simulink library "RF"  (Simulink 4.00)
values from neighbouring files (symbols this model uses):
  A = rms(interp1(f,MX,fb))    [fftbandamp.m]    (also in logfft.m = fftamp(samples, fs, f, varargin{:})/vpp; plotfft.m = fftamp(samples, fs, f, varargin{:})*2/vpp)
  P = sinc((1575.42 - f)/10.23).^2./10.23    [L1PSD.m]    (also in fftphase.m = interp1(f,PX,f0))
undefined symbols (not defined in the file or in its folder): adb, B, CA_ID, fs, j, m, N, p, Phi, Range, Rice_K, Rice_Seed, Rice_Sigma, tau_delay, z
libraries: RF x133, dspcmplx x47, com_sour x8, dspelmat x8, com_chan x4, dspbdsp x3, dspswit x3, simulink_extras x2, com_filt x2
(part 5 of 5)

== system RF/GPS Blocks/C/A Code, 1.023MHz/PN1/1-step delay9 ==
  in_1 : Inport  Port=1
  Constant : Constant  Value=ini
  Constant1 : Constant  Value=n*ts(1)+ts(2)
  Digital Clock : DigitalClock  SampleTime=ts
  K-step delay : DiscreteFilter  Numerator=[zeros(1,n), 1]  Denominator=1  SampleTime=ts  Realization=auto
  Relational Operator : RelationalOperator  Operator=>=
  Switch : Switch  Threshold=.1
  out_1 : Outport  Port=1  InitialOutput=0
  wires:
  Relational Operator/1 -> Switch/2
  Constant1/1 -> Relational Operator/2
  Digital Clock/1 -> Relational Operator/1
  Constant/1 -> Switch/3
  K-step delay/1 -> Switch/1
  in_1/1 -> K-step delay/1
  Switch/1 -> out_1/1

== system RF/GPS Blocks/C/A Code, 1.023MHz/PN2/1-step delay1 ==
  in_1 : Inport  Port=1
  Constant : Constant  Value=ini
  Constant1 : Constant  Value=n*ts(1)+ts(2)
  Digital Clock : DigitalClock  SampleTime=ts
  K-step delay : DiscreteFilter  Numerator=[zeros(1,n), 1]  Denominator=1  SampleTime=ts  Realization=auto
  Relational Operator : RelationalOperator  Operator=>=
  Switch : Switch  Threshold=.1
  out_1 : Outport  Port=1  InitialOutput=0
  wires:
  Relational Operator/1 -> Switch/2
  Constant1/1 -> Relational Operator/2
  Digital Clock/1 -> Relational Operator/1
  Constant/1 -> Switch/3
  K-step delay/1 -> Switch/1
  in_1/1 -> K-step delay/1
  Switch/1 -> out_1/1

== system RF/GPS Blocks/C/A Code, 1.023MHz/PN2/1-step delay10 ==
  in_1 : Inport  Port=1
  Constant : Constant  Value=ini
  Constant1 : Constant  Value=n*ts(1)+ts(2)
  Digital Clock : DigitalClock  SampleTime=ts
  K-step delay : DiscreteFilter  Numerator=[zeros(1,n), 1]  Denominator=1  SampleTime=ts  Realization=auto
  Relational Operator : RelationalOperator  Operator=>=
  Switch : Switch  Threshold=.1
  out_1 : Outport  Port=1  InitialOutput=0
  wires:
  Relational Operator/1 -> Switch/2
  Constant1/1 -> Relational Operator/2
  Digital Clock/1 -> Relational Operator/1
  Constant/1 -> Switch/3
  K-step delay/1 -> Switch/1
  in_1/1 -> K-step delay/1
  Switch/1 -> out_1/1

== system RF/GPS Blocks/C/A Code, 1.023MHz/PN2/1-step delay2 ==
  in_1 : Inport  Port=1
  Constant : Constant  Value=ini
  Constant1 : Constant  Value=n*ts(1)+ts(2)
  Digital Clock : DigitalClock  SampleTime=ts
  K-step delay : DiscreteFilter  Numerator=[zeros(1,n), 1]  Denominator=1  SampleTime=ts  Realization=auto
  Relational Operator : RelationalOperator  Operator=>=
  Switch : Switch  Threshold=.1
  out_1 : Outport  Port=1  InitialOutput=0
  wires:
  Relational Operator/1 -> Switch/2
  Constant1/1 -> Relational Operator/2
  Digital Clock/1 -> Relational Operator/1
  Constant/1 -> Switch/3
  K-step delay/1 -> Switch/1
  in_1/1 -> K-step delay/1
  Switch/1 -> out_1/1

== system RF/GPS Blocks/C/A Code, 1.023MHz/PN2/1-step delay3 ==
  in_1 : Inport  Port=1
  Constant : Constant  Value=ini
  Constant1 : Constant  Value=n*ts(1)+ts(2)
  Digital Clock : DigitalClock  SampleTime=ts
  K-step delay : DiscreteFilter  Numerator=[zeros(1,n), 1]  Denominator=1  SampleTime=ts  Realization=auto
  Relational Operator : RelationalOperator  Operator=>=
  Switch : Switch  Threshold=.1
  out_1 : Outport  Port=1  InitialOutput=0
  wires:
  Relational Operator/1 -> Switch/2
  Constant1/1 -> Relational Operator/2
  Digital Clock/1 -> Relational Operator/1
  Constant/1 -> Switch/3
  K-step delay/1 -> Switch/1
  in_1/1 -> K-step delay/1
  Switch/1 -> out_1/1

== system RF/GPS Blocks/C/A Code, 1.023MHz/PN2/1-step delay4 ==
  in_1 : Inport  Port=1
  Constant : Constant  Value=ini
  Constant1 : Constant  Value=n*ts(1)+ts(2)
  Digital Clock : DigitalClock  SampleTime=ts
  K-step delay : DiscreteFilter  Numerator=[zeros(1,n), 1]  Denominator=1  SampleTime=ts  Realization=auto
  Relational Operator : RelationalOperator  Operator=>=
  Switch : Switch  Threshold=.1
  out_1 : Outport  Port=1  InitialOutput=0
  wires:
  Relational Operator/1 -> Switch/2
  Constant1/1 -> Relational Operator/2
  Digital Clock/1 -> Relational Operator/1
  Constant/1 -> Switch/3
  K-step delay/1 -> Switch/1
  in_1/1 -> K-step delay/1
  Switch/1 -> out_1/1

== system RF/GPS Blocks/C/A Code, 1.023MHz/PN2/1-step delay5 ==
  in_1 : Inport  Port=1
  Constant : Constant  Value=ini
  Constant1 : Constant  Value=n*ts(1)+ts(2)
  Digital Clock : DigitalClock  SampleTime=ts
  K-step delay : DiscreteFilter  Numerator=[zeros(1,n), 1]  Denominator=1  SampleTime=ts  Realization=auto
  Relational Operator : RelationalOperator  Operator=>=
  Switch : Switch  Threshold=.1
  out_1 : Outport  Port=1  InitialOutput=0
  wires:
  Relational Operator/1 -> Switch/2
  Constant1/1 -> Relational Operator/2
  Digital Clock/1 -> Relational Operator/1
  Constant/1 -> Switch/3
  K-step delay/1 -> Switch/1
  in_1/1 -> K-step delay/1
  Switch/1 -> out_1/1

== system RF/GPS Blocks/C/A Code, 1.023MHz/PN2/1-step delay6 ==
  in_1 : Inport  Port=1
  Constant : Constant  Value=ini
  Constant1 : Constant  Value=n*ts(1)+ts(2)
  Digital Clock : DigitalClock  SampleTime=ts
  K-step delay : DiscreteFilter  Numerator=[zeros(1,n), 1]  Denominator=1  SampleTime=ts  Realization=auto
  Relational Operator : RelationalOperator  Operator=>=
  Switch : Switch  Threshold=.1
  out_1 : Outport  Port=1  InitialOutput=0
  wires:
  Relational Operator/1 -> Switch/2
  Constant1/1 -> Relational Operator/2
  Digital Clock/1 -> Relational Operator/1
  Constant/1 -> Switch/3
  K-step delay/1 -> Switch/1
  in_1/1 -> K-step delay/1
  Switch/1 -> out_1/1

== system RF/GPS Blocks/C/A Code, 1.023MHz/PN2/1-step delay7 ==
  in_1 : Inport  Port=1
  Constant : Constant  Value=ini
  Constant1 : Constant  Value=n*ts(1)+ts(2)
  Digital Clock : DigitalClock  SampleTime=ts
  K-step delay : DiscreteFilter  Numerator=[zeros(1,n), 1]  Denominator=1  SampleTime=ts  Realization=auto
  Relational Operator : RelationalOperator  Operator=>=
  Switch : Switch  Threshold=.1
  out_1 : Outport  Port=1  InitialOutput=0
  wires:
  Relational Operator/1 -> Switch/2
  Constant1/1 -> Relational Operator/2
  Digital Clock/1 -> Relational Operator/1
  Constant/1 -> Switch/3
  K-step delay/1 -> Switch/1
  in_1/1 -> K-step delay/1
  Switch/1 -> out_1/1

== system RF/GPS Blocks/C/A Code, 1.023MHz/PN2/1-step delay8 ==
  in_1 : Inport  Port=1
  Constant : Constant  Value=ini
  Constant1 : Constant  Value=n*ts(1)+ts(2)
  Digital Clock : DigitalClock  SampleTime=ts
  K-step delay : DiscreteFilter  Numerator=[zeros(1,n), 1]  Denominator=1  SampleTime=ts  Realization=auto
  Relational Operator : RelationalOperator  Operator=>=
  Switch : Switch  Threshold=.1
  out_1 : Outport  Port=1  InitialOutput=0
  wires:
  Relational Operator/1 -> Switch/2
  Constant1/1 -> Relational Operator/2
  Digital Clock/1 -> Relational Operator/1
  Constant/1 -> Switch/3
  K-step delay/1 -> Switch/1
  in_1/1 -> K-step delay/1
  Switch/1 -> out_1/1

== system RF/GPS Blocks/C/A Code, 1.023MHz/PN2/1-step delay9 ==
  in_1 : Inport  Port=1
  Constant : Constant  Value=ini
  Constant1 : Constant  Value=n*ts(1)+ts(2)
  Digital Clock : DigitalClock  SampleTime=ts
  K-step delay : DiscreteFilter  Numerator=[zeros(1,n), 1]  Denominator=1  SampleTime=ts  Realization=auto
  Relational Operator : RelationalOperator  Operator=>=
  Switch : Switch  Threshold=.1
  out_1 : Outport  Port=1  InitialOutput=0
  wires:
  Relational Operator/1 -> Switch/2
  Constant1/1 -> Relational Operator/2
  Digital Clock/1 -> Relational Operator/1
  Constant/1 -> Switch/3
  K-step delay/1 -> Switch/1
  in_1/1 -> K-step delay/1
  Switch/1 -> out_1/1

== system RF/GPS Blocks/GPS Channel/AWGN channel/Gaussian noise generator1 ==
  Constant : Constant  Value=m
  Matrix Gain : StateSpace  A=[]  B=[]  C=[]  D=K  X0=0  Realization=auto  AbsoluteTolerance=auto  mask(Matrix Gain){@1=d}
      mask prompts: @1 "Gain matrix:"
      mask help: Matrix Gain.
      mask init:
      | K = @1;
      mask Help: Multiplies input vector by entered matrix to produce output vector (y=Au).
      mask Display: disp('K')
  Random Number : RandomNumber  Mean=0  Variance=1  Seed=s  SampleTime=-1
  Sum : Sum  Inputs=++  SaturateOnIntegerOverflow=on
  out_1 : Outport  Port=1  InitialOutput=0
  wires:
  Constant/1 -> Sum/1
  Random Number/1 -> Matrix Gain/1
  Matrix Gain/1 -> Sum/2
  Sum/1 -> out_1/1

== system RF/GPS Blocks/GPS Transmitter/BPSK mod, 1575MHz1/MPSK map ==
  in_1 : Inport  Port=1
  Multiple factor : Constant  Value=Sft
  Product : Product  Inputs=2  Multiplication=Element-wise(.*)  SaturateOnIntegerOverflow=on
  Zero-Order Hold1 : ZeroOrderHold  SampleTime=td
  out_1 : Outport  Port=1  InitialOutput=0
  wires:
  Zero-Order Hold1/1 -> Product/1
  in_1/1 -> Zero-Order Hold1/1
  Product/1 -> out_1/1
  Multiple factor/1 -> Product/2

== system RF/GPS Blocks/GPS Transmitter/BPSK mod, 1575MHz1/PM passband ==
  in_1 : Inport  Port=1  SampleTime=ts
  Clock : Clock
      settings: DisplayTime=off  Decimation=10
  Fcn : Fcn  Expr=cos(u[1])
  Gain : Gain  Gain=Fc  Multiplication=Element-wise(K.*u)  SaturateOnIntegerOverflow=on
  Initial value : Constant  Value=Ph
  Sum1 : Sum  Inputs=+++  SaturateOnIntegerOverflow=on
  Sum2 : Sum  Inputs=+-  SaturateOnIntegerOverflow=on
  Zero-Order Hold : ZeroOrderHold  SampleTime=td
  out_1 : Outport  Port=1  InitialOutput=0
  wires:
  Fcn/1 -> out_1/1
  Initial value/1 -> Sum1/3
  Sum1/1 -> Fcn/1
  in_1/1 -> Sum1/1
  Clock/1 -> Gain/1
  Sum2/1 -> Sum1/2
  Zero-Order Hold/1 -> Sum2/2
  Gain/1 -> Sum2/1, Zero-Order Hold/1

== system RF/GPS Blocks/GPS Transmitter/BPSK mod, 1575MHz2/MPSK map ==
  in_1 : Inport  Port=1
  Multiple factor : Constant  Value=Sft
  Product : Product  Inputs=2  Multiplication=Element-wise(.*)  SaturateOnIntegerOverflow=on
  Zero-Order Hold1 : ZeroOrderHold  SampleTime=td
  out_1 : Outport  Port=1  InitialOutput=0
  wires:
  Zero-Order Hold1/1 -> Product/1
  in_1/1 -> Zero-Order Hold1/1
  Product/1 -> out_1/1
  Multiple factor/1 -> Product/2

== system RF/GPS Blocks/GPS Transmitter/BPSK mod, 1575MHz2/PM passband ==
  in_1 : Inport  Port=1  SampleTime=ts
  Clock : Clock
      settings: DisplayTime=off  Decimation=10
  Fcn : Fcn  Expr=cos(u[1])
  Gain : Gain  Gain=Fc  Multiplication=Element-wise(K.*u)  SaturateOnIntegerOverflow=on
  Initial value : Constant  Value=Ph
  Sum1 : Sum  Inputs=+++  SaturateOnIntegerOverflow=on
  Sum2 : Sum  Inputs=+-  SaturateOnIntegerOverflow=on
  Zero-Order Hold : ZeroOrderHold  SampleTime=td
  out_1 : Outport  Port=1  InitialOutput=0
  wires:
  Fcn/1 -> out_1/1
  Initial value/1 -> Sum1/3
  Sum1/1 -> Fcn/1
  in_1/1 -> Sum1/1
  Clock/1 -> Gain/1
  Sum2/1 -> Sum1/2
  Zero-Order Hold/1 -> Sum2/2
  Gain/1 -> Sum2/1, Zero-Order Hold/1

== system RF/GPS Blocks/GPS Transmitter/P Code, 10.23MHz/P Code, 10.23MHz ==
  Uniform number : S-Function  FunctionName=srandint  Parameters=seed,mul  PortCounts=[]  SFunctionModules=''
  out_1 : Outport  Port=1  InitialOutput=0
  wires:
  Uniform number/1 -> out_1/1

== system RF/Transmission  Channel Blocks/Doppler Fading Envelope/FFT Filter4/Buffer ==
  in_1 : Inport  Port=1
  Buffer : S-Function  FunctionName=sbufferc  Parameters=N,V,Ts,ic  PortCounts=[]  SFunctionModules=''
  ZOH : S-Function  FunctionName=szoh  Parameters=Ts*(N-V)  PortCounts=[]  SFunctionModules=''
  Zero-Order Hold : ZeroOrderHold  SampleTime=Ts
  Outport : Outport  Port=1  InitialOutput=0
  wires:
  Zero-Order Hold/1 -> Buffer/1
  in_1/1 -> Zero-Order Hold/1
  ZOH/1 -> Outport/1
  Buffer/1 -> ZOH/1

== system RF/Transmission  Channel Blocks/Doppler Fading Envelope/FFT Filter4/Complex Multiply1 ==
  note: R = Real
      | I = Imaginary
  Complex input 1 : Inport  Port=1
  Complex input 2 : Inport  Port=2
  Join : dspcmplx/Join
  Product{,1..3} (4 alike) : Product  Inputs=2  Multiplication=Element-wise(.*)  SaturateOnIntegerOverflow=on
  Split : dspcmplx/Split
  Split1 : dspcmplx/Split
  Sum : Sum  Inputs=+-  SaturateOnIntegerOverflow=on
  Sum1 : Sum  Inputs=++  SaturateOnIntegerOverflow=on
  Complex Multiply Result : Outport  Port=1  InitialOutput=0
  wires:
  Product2/1 -> Sum1/2
  Product3/1 -> Sum1/1
  Split/2 -> Product1/1, Product2/2  "I1"
  Split1/2 -> Product1/2, Product3/2  "I2"
  Split1/1 -> Product/2, Product2/1  "R2"
  Split/1 -> Product/1, Product3/1  "R1"
  Product1/1 -> Sum/2
  Product/1 -> Sum/1
  Complex input 2/1 -> Split1/1
  Complex input 1/1 -> Split/1
  Sum/1 -> Join/1  "Rout"
  Sum1/1 -> Join/2  "Iout"
  Join/1 -> Complex Multiply Result/1

== system RF/Transmission  Channel Blocks/Doppler Fading Envelope/FFT Filter4/Filter Response ==
  Complex Constant : Constant  Value=C
  Out1 : Outport  Port=1  InitialOutput=0
  wires:
  Complex Constant/1 -> Out1/1

== system RF/Transmission  Channel Blocks/Doppler Fading Envelope/FFT Filter4/Partial Unbuffer ==
  in_1 : Inport  Port=1
  Complete Unbuffer : S-Function  FunctionName=sunbuffc  Parameters=num_chans,Ts  PortCounts=[]  SFunctionModules=''
  Selector : Selector  InputType=Vector  ElementSrc=Internal  Elements=elements  RowSrc=Internal  Rows=1  ColumnSrc=Internal  Columns=1  InputPortWidth=N*num_chans
  ZOH : S-Function  FunctionName=szoh  Parameters=Ts  PortCounts=[]  SFunctionModules=''
  out_1 : Outport  Port=1  InitialOutput=0
  wires:
  in_1/1 -> Selector/1
  Selector/1 -> ZOH/1
  ZOH/1 -> Complete Unbuffer/1
  Complete Unbuffer/1 -> out_1/1

== system RF/Transmission  Channel Blocks/Doppler Fading Envelope/FFT Filter4/Real FFT ==
  in_1 : Inport  Port=1
  FFT(u) : S-Function  FunctionName=srfftc  Parameters=-1  PortCounts=[]  SFunctionModules='fft'
  out_1 : Outport  Port=1  InitialOutput=0
  wires:
  FFT(u)/1 -> out_1/1
  in_1/1 -> FFT(u)/1

== system RF/Transmission  Channel Blocks/Doppler Fading Envelope/FFT Filter4/Real IFFT ==
  in_1 : Inport  Port=1
  IFFT : S-Function  FunctionName=srifft  Parameters=-1  PortCounts=[]  SFunctionModules='fft'
  Real : dspcmplx/Real
  out_1 : Outport  Port=1  InitialOutput=0
  wires:
  IFFT/1 -> Real/1
  Real/1 -> out_1/1
  in_1/1 -> IFFT/1

== system RF/Transmission  Channel Blocks/Doppler Fading Envelope/FFT Filter5/Buffer ==
  in_1 : Inport  Port=1
  Buffer : S-Function  FunctionName=sbufferc  Parameters=N,V,Ts,ic  PortCounts=[]  SFunctionModules=''
  ZOH : S-Function  FunctionName=szoh  Parameters=Ts*(N-V)  PortCounts=[]  SFunctionModules=''
  Zero-Order Hold : ZeroOrderHold  SampleTime=Ts
  Outport : Outport  Port=1  InitialOutput=0
  wires:
  Zero-Order Hold/1 -> Buffer/1
  in_1/1 -> Zero-Order Hold/1
  ZOH/1 -> Outport/1
  Buffer/1 -> ZOH/1

== system RF/Transmission  Channel Blocks/Doppler Fading Envelope/FFT Filter5/Complex Multiply1 ==
  note: R = Real
      | I = Imaginary
  Complex input 1 : Inport  Port=1
  Complex input 2 : Inport  Port=2
  Join : dspcmplx/Join
  Product{,1..3} (4 alike) : Product  Inputs=2  Multiplication=Element-wise(.*)  SaturateOnIntegerOverflow=on
  Split : dspcmplx/Split
  Split1 : dspcmplx/Split
  Sum : Sum  Inputs=+-  SaturateOnIntegerOverflow=on
  Sum1 : Sum  Inputs=++  SaturateOnIntegerOverflow=on
  Complex Multiply Result : Outport  Port=1  InitialOutput=0
  wires:
  Product2/1 -> Sum1/2
  Product3/1 -> Sum1/1
  Split/2 -> Product1/1, Product2/2  "I1"
  Split1/2 -> Product1/2, Product3/2  "I2"
  Split1/1 -> Product/2, Product2/1  "R2"
  Split/1 -> Product/1, Product3/1  "R1"
  Product1/1 -> Sum/2
  Product/1 -> Sum/1
  Complex input 2/1 -> Split1/1
  Complex input 1/1 -> Split/1
  Sum/1 -> Join/1  "Rout"
  Sum1/1 -> Join/2  "Iout"
  Join/1 -> Complex Multiply Result/1

== system RF/Transmission  Channel Blocks/Doppler Fading Envelope/FFT Filter5/Filter Response ==
  Complex Constant : Constant  Value=C
  Out1 : Outport  Port=1  InitialOutput=0
  wires:
  Complex Constant/1 -> Out1/1

== system RF/Transmission  Channel Blocks/Doppler Fading Envelope/FFT Filter5/Partial Unbuffer ==
  in_1 : Inport  Port=1
  Complete Unbuffer : S-Function  FunctionName=sunbuffc  Parameters=num_chans,Ts  PortCounts=[]  SFunctionModules=''
  Selector : Selector  InputType=Vector  ElementSrc=Internal  Elements=elements  RowSrc=Internal  Rows=1  ColumnSrc=Internal  Columns=1  InputPortWidth=N*num_chans
  ZOH : S-Function  FunctionName=szoh  Parameters=Ts  PortCounts=[]  SFunctionModules=''
  out_1 : Outport  Port=1  InitialOutput=0
  wires:
  in_1/1 -> Selector/1
  Selector/1 -> ZOH/1
  ZOH/1 -> Complete Unbuffer/1
  Complete Unbuffer/1 -> out_1/1

== system RF/Transmission  Channel Blocks/Doppler Fading Envelope/FFT Filter5/Real FFT ==
  in_1 : Inport  Port=1
  FFT(u) : S-Function  FunctionName=srfftc  Parameters=-1  PortCounts=[]  SFunctionModules='fft'
  out_1 : Outport  Port=1  InitialOutput=0
  wires:
  FFT(u)/1 -> out_1/1
  in_1/1 -> FFT(u)/1

== system RF/Transmission  Channel Blocks/Doppler Fading Envelope/FFT Filter5/Real IFFT ==
  in_1 : Inport  Port=1
  IFFT : S-Function  FunctionName=srifft  Parameters=-1  PortCounts=[]  SFunctionModules='fft'
  Real : dspcmplx/Real
  out_1 : Outport  Port=1  InitialOutput=0
  wires:
  IFFT/1 -> Real/1
  Real/1 -> out_1/1
  in_1/1 -> IFFT/1
